simulink model "Motor_doble_debanado"  (R2020b)
settings: Solver=VariableStepAuto  StartTime=0.0  StopTime=3  RelTol=1e-3
values from neighbouring files (symbols this model uses):
  C0 = 0.05    [Motor_doble_devanado.m]
  J = 0.016    [Motor_doble_devanado.m]
  Lr = 0.1    [Motor_doble_devanado.m]
  Ls = 0.1    [Motor_doble_devanado.m]
  M = 0.05    [Motor_doble_devanado.m]
  Rr = 0.5    [Motor_doble_devanado.m]
  Rs = 10    [Motor_doble_devanado.m]
  Tload = 2    [Motor_doble_devanado.m]
  V = 180    [Motor_doble_devanado.m]
settings Model: Creator=diego  LastModifiedBy=diego

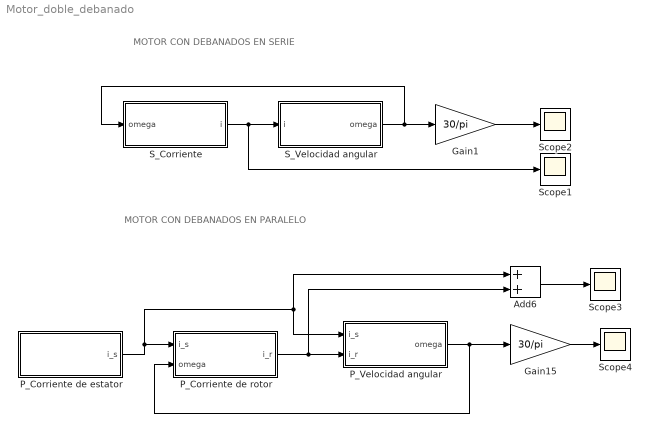
== system Motor_doble_debanado ==
  note: MOTOR CON DEBANADOS EN SERIE
  note: MOTOR CON DEBANADOS EN PARALELO
  Add6 : Sum
  Gain1 : Gain  Gain=30/pi
  Gain15 : Gain  Gain=30/pi
  P_Corriente de estator : Subsystem
  P_Corriente de rotor : Subsystem
  P_Velocidad angular : Subsystem
  S_Corriente : Subsystem
  S_Velocidad angular : Subsystem
  Scope{1..4} (4 alike) : Scope
  wires:
  P_Corriente de estator/1(i_s) -> P_Velocidad angular/1(i_s), Add6/1, P_Corriente de rotor/1(i_s)
  P_Corriente de rotor/1(i_r) -> Add6/2, P_Velocidad angular/2(i_r)
  P_Velocidad angular/1(omega) -> Gain15/1, P_Corriente de rotor/2(omega)
  Add6/1 -> Scope3/1
  Gain15/1 -> Scope4/1
  S_Corriente/1(i) -> Scope1/1, S_Velocidad angular/1(i)
  Gain1/1 -> Scope2/1
  S_Velocidad angular/1(omega) -> Gain1/1, S_Corriente/1(omega)

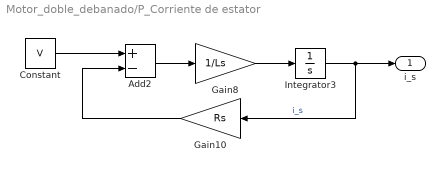
== system Motor_doble_debanado/P_Corriente de estator ==
  Add2 : Sum  Inputs=+-
  Constant : Constant  Value=V
  Gain10 : Gain  Gain=Rs
  Gain8 : Gain  Gain=1/Ls
  Integrator3 : Integrator
  i_s : Outport
  wires:
  Gain10/1 -> Add2/2
  Gain8/1 -> Integrator3/1
  Integrator3/1 -> i_s/1, Gain10/1  "i_s"
  Add2/1 -> Gain8/1
  Constant/1 -> Add2/1

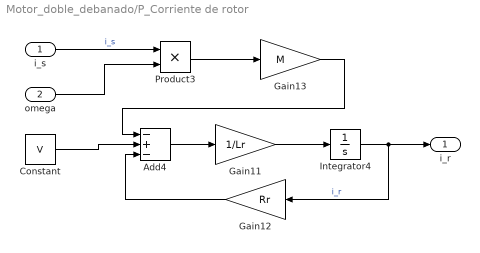
== system Motor_doble_debanado/P_Corriente de rotor ==
  i_s : Inport
  omega : Inport  Port=2
  Add4 : Sum  Inputs=-+-
  Constant : Constant  Value=V
  Gain11 : Gain  Gain=1/Lr
  Gain12 : Gain  Gain=Rr
  Gain13 : Gain  Gain=M
  Integrator4 : Integrator
  Product3 : Product
  i_r : Outport
  wires:
  i_s/1 -> Product3/1  "i_s"
  Add4/1 -> Gain11/1
  Integrator4/1 -> i_r/1, Gain12/1  "i_r"
  Gain11/1 -> Integrator4/1
  Gain13/1 -> Add4/1
  Gain12/1 -> Add4/3
  Product3/1 -> Gain13/1
  omega/1 -> Product3/2
  Constant/1 -> Add4/2

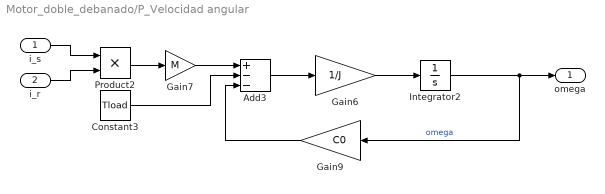
== system Motor_doble_debanado/P_Velocidad angular ==
  i_s : Inport
  i_r : Inport  Port=2
  Add3 : Sum  Inputs=+--
  Constant3 : Constant  Value=Tload
  Gain6 : Gain  Gain=1/J
  Gain7 : Gain  Gain=M
  Gain9 : Gain  Gain=C0
  Integrator2 : Integrator
  Product2 : Product
  omega : Outport
  wires:
  Constant3/1 -> Add3/2
  Integrator2/1 -> omega/1, Gain9/1  "omega"
  Gain6/1 -> Integrator2/1
  Gain7/1 -> Add3/1
  Add3/1 -> Gain6/1
  Gain9/1 -> Add3/3
  Product2/1 -> Gain7/1
  i_s/1 -> Product2/1
  i_r/1 -> Product2/2

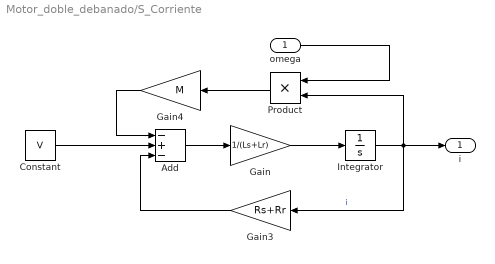
== system Motor_doble_debanado/S_Corriente ==
  omega : Inport
  Add : Sum  Inputs=-+-
  Constant : Constant  Value=V
  Gain : Gain  Gain=1/(Ls+Lr)
  Gain3 : Gain  Gain=Rs+Rr
  Gain4 : Gain  Gain=M
  Integrator : Integrator
  Product : Product
  i : Outport
  wires:
  Gain3/1 -> Add/3
  Constant/1 -> Add/2
  Integrator/1 -> Product/2, i/1, Gain3/1  "i"
  Gain4/1 -> Add/1
  Gain/1 -> Integrator/1
  Add/1 -> Gain/1
  omega/1 -> Product/1
  Product/1 -> Gain4/1

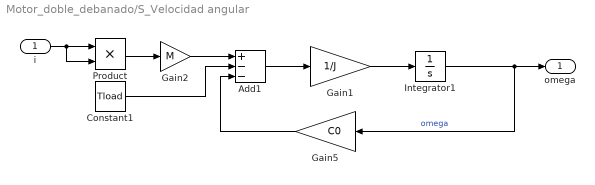
== system Motor_doble_debanado/S_Velocidad angular ==
  i : Inport
  Add1 : Sum  Inputs=+--
  Constant1 : Constant  Value=Tload
  Gain1 : Gain  Gain=1/J
  Gain2 : Gain  Gain=M
  Gain5 : Gain  Gain=C0
  Integrator1 : Integrator
  Product : Product
  omega : Outport
  wires:
  Gain5/1 -> Add1/3
  Constant1/1 -> Add1/2
  Product/1 -> Gain2/1
  Add1/1 -> Gain1/1
  Integrator1/1 -> omega/1, Gain5/1  "omega"
  Gain1/1 -> Integrator1/1
  Gain2/1 -> Add1/1
  i/1 -> Product/2, Product/1
